simulink model "s_abeob2"  (Simulink 2.00)
settings: Solver=ode45  StartTime=0.0  StopTime=20  MaxStep=0.10  RelTol=1e-3  AbsTol=1e-6
values from neighbouring files (symbols this model uses):
  Cd = C    [abeob1.m]    (also in akalm1.m; kalm2.m; kalm3.m; kalm4.m)
  F = K*(x_un/x_un(1))/kq1    [abeob1.m]    (also in akalm1.m = xp_un*alpha; alqr1.m = K*(x_un/x_un(1))/k1; alqrd1.m = K*(x_un/x_un(1))/k1; apol1.m = K*(x_un/x_un(1))/k1)
  kq1 = K(1)    [abeob1.m]
  Ts = 0.5    [abeob1.m]    (also in akalm1.m = 0.25; alqrd1.m = 0.25; kalm2.m; kalm3.m)
  x0 = [5, 0, 0, 0]    [abeob1.m]    (also in alqr1.m; alqrd1.m; apol1.m; estimate_1.m = [1 2 3])
settings Model: SaveTime=off  SaveOutput=off  ConsistencyChecking=off

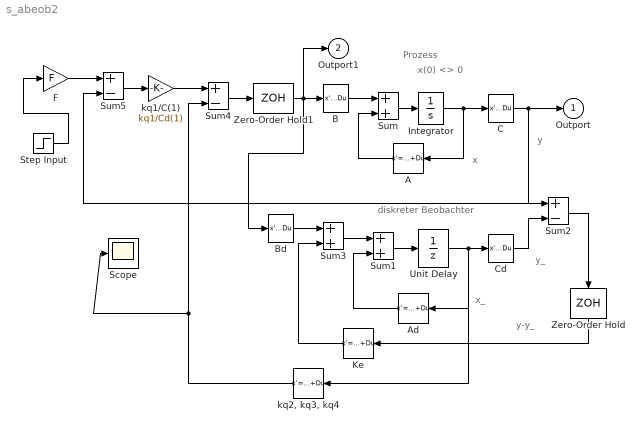
== system s_abeob2 ==
  note: y_
  note: Prozess
  note: x(0) <> 0
  note: y
  note: diskreter Beobachter
  note: x_
  note: x
  note: y-y_
  " kq2, kq3, kq4" : StateSpace  Orientation=left  A=[]  B=[]  C=[]  D=K  X0=0  mask(Matrix Gain){@1=[0 kq2 kq3 kq4]}
      mask prompts: @1 "Gain matrix:"
      mask help: Matrix Gain.
      mask init:
      | K = @1;
      mask Help: Multiplies input vector by entered matrix to produce output vector (y=Au).
      mask Display: disp('K')
  A : StateSpace  Orientation=left  A=[]  B=[]  C=[]  D=K  X0=0  mask(Matrix Gain){@1=A}
      mask prompts: @1 "Gain matrix:"
      mask help: Matrix Gain.
      mask init:
      | K = @1;
      mask Help: Multiplies input vector by entered matrix to produce output vector (y=Au).
      mask Display: disp('K')
  Ad : StateSpace  Orientation=left  A=[]  B=[]  C=[]  D=K  X0=0  mask(Matrix Gain){@1=Ad}
      mask prompts: @1 "Gain matrix:"
      mask help: Matrix Gain.
      mask init:
      | K = @1;
      mask Help: Multiplies input vector by entered matrix to produce output vector (y=Au).
      mask Display: disp('K')
  B : StateSpace  A=[]  B=[]  C=[]  D=K  X0=0  mask(Matrix Gain){@1=B}
      mask prompts: @1 "Gain matrix:"
      mask help: Matrix Gain.
      mask init:
      | K = @1;
      mask Help: Multiplies input vector by entered matrix to produce output vector (y=Au).
      mask Display: disp('K')
  Bd : StateSpace  A=[]  B=[]  C=[]  D=K  X0=0  mask(Matrix Gain){@1=Bd}
      mask prompts: @1 "Gain matrix:"
      mask help: Matrix Gain.
      mask init:
      | K = @1;
      mask Help: Multiplies input vector by entered matrix to produce output vector (y=Au).
      mask Display: disp('K')
  C : StateSpace  A=[]  B=[]  C=[]  D=K  X0=0  mask(Matrix Gain){@1=C}
      mask prompts: @1 "Gain matrix:"
      mask help: Matrix Gain.
      mask init:
      | K = @1;
      mask Help: Multiplies input vector by entered matrix to produce output vector (y=Au).
      mask Display: disp('K')
  Cd : StateSpace  A=[]  B=[]  C=[]  D=K  X0=0  mask(Matrix Gain){@1=Cd}
      mask prompts: @1 "Gain matrix:"
      mask help: Matrix Gain.
      mask init:
      | K = @1;
      mask Help: Multiplies input vector by entered matrix to produce output vector (y=Au).
      mask Display: disp('K')
  F : Gain  Gain=F
  Integrator : Integrator  ExternalReset=none  InitialConditionSource=internal  InitialCondition=[x0]  LimitOutput=off  UpperSaturationLimit=inf  LowerSaturationLimit=-inf  ShowSaturationPort=off  ShowStatePort=off  AbsoluteTolerance=auto
  Ke : StateSpace  Orientation=left  A=[]  B=[]  C=[]  D=K  X0=0  mask(Matrix Gain){@1=Ke}
      mask prompts: @1 "Gain matrix:"
      mask help: Matrix Gain.
      mask init:
      | K = @1;
      mask Help: Multiplies input vector by entered matrix to produce output vector (y=Au).
      mask Display: disp('K')
  Scope : Scope
      settings: TickLabels=on  TimeRange=23.600000  YMin=-12.600000  YMax=12.600000  SaveToWorkspace=off  SaveName=ScopeData
  Step Input : Step  Time=2.5  Before=0  After=1
  Sum : Sum  Inputs=++
  Sum1 : Sum  Inputs=++
  Sum2 : Sum  Inputs=+-
  Sum3 : Sum  Inputs=++
  Sum4 : Sum  Inputs=+-
  Sum5 : Sum  Inputs=+-
  Unit Delay : UnitDelay  X0=0  SampleTime=Ts
  Zero-Order Hold : ZeroOrderHold  Orientation=down  SampleTime=Ts
  Zero-Order Hold1 : ZeroOrderHold  SampleTime=Ts
  kq1/C(1) : Gain  Gain=kq1/Cd(1)
  Outport : Outport  Port=1  InitialOutput=0
  Outport1 : Outport  Port=2  InitialOutput=0
  wires:
  " kq2, kq3, kq4"/1 -> Scope/1, Sum4/2
  C/1 -> Sum5/2, Outport/1, Sum2/1
  Zero-Order Hold1/1 -> Outport1/1, Bd/1, B/1
  Sum4/1 -> Zero-Order Hold1/1
  Step Input/1 -> F/1
  F/1 -> Sum5/1
  Sum5/1 -> kq1/C(1)/1
  kq1/C(1)/1 -> Sum4/1
  Unit Delay/1 -> " kq2, kq3, kq4"/1, Cd/1, Ad/1
  Zero-Order Hold/1 -> Ke/1
  Sum2/1 -> Zero-Order Hold/1
  Bd/1 -> Sum3/1
  Ke/1 -> Sum3/2
  Sum3/1 -> Sum1/1
  Cd/1 -> Sum2/2
  Ad/1 -> Sum1/2
  Sum1/1 -> Unit Delay/1
  Integrator/1 -> C/1, A/1
  A/1 -> Sum/2
  Sum/1 -> Integrator/1
  B/1 -> Sum/1
